simulink model "hover_model_estim_bsc_simple_v15"  (Simulink 7.1)
settings: Solver=ode45  StartTime=0.0  StopTime=200  RelTol=1e-4
values from neighbouring files (symbols this model uses):
  Am = [0 1 0 0 0 0;     0 0 0 0 0 0;     0 0 0 1 0 0;     0 0 0 0 0 0;     0 0 0 0 0 1;     0 0 0 0 0 0]    [Hover.m]    (also in Hoverparameter1.m = [0,1;0,0])
  Bm = [0 0 0 0;     -Kt/Jy -Kt/Jy Kt/Jy Kt/Jy;     0 0 0 0;     I*Kfn/Jp -I*Kfn/Jp 0 0;     0 0 0 0;     0 0 I*Kfc/Jr -I*Kfc/Jr]    [Hover.m]    (also in Hoverparameter1.m = [0,0,0,0;1,-1,0,0])
  Cm = [1 0 0 0 0 0;     0 0 1 0 0 0;     0 0 0 0 1 0]    [Hover.m]    (also in Hoverparameter1.m = [1,0])
  Ki = K(:,7:9)    [Hover.m]    (also in Hoverparameter1.m)
libraries: simulink x5, vrlib x1, simulink_extras x1
settings Model: Creator=user  LastModifiedBy=MorrisChen
settings DataIOCC: SignalLoggingName=sigsOut
settings OptimizationCC: InlineInvariantSignals=on
settings DebuggingCC: SaveWithParameterizedLinksMsg=none  SignalResolutionControl=TryResolveAllWithWarning  SolverPrmCheckMsg=none  MultiTaskDSMMsg=warning  MultiTaskCondExecSysMsg=none  StrictBusMsg=None
settings HardwareCC: TargetUnknown=on
settings RTWCC: IncludeERTFirstTime=on
settings GRTTargetCC: TargetFcnLib=ansi_tfl_tmw.mat

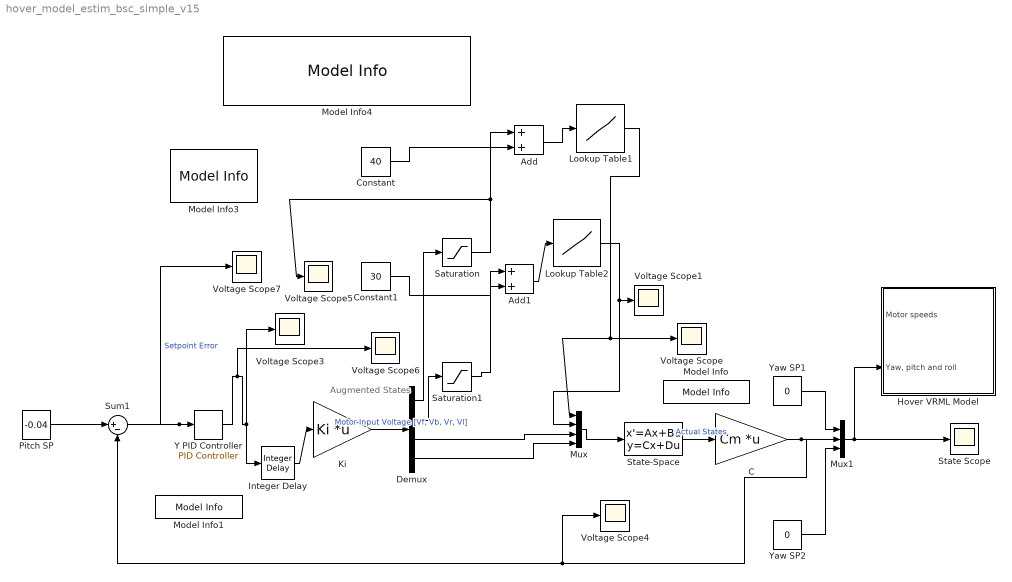
== system hover_model_estim_bsc_simple_v15 ==
  note: Augmented
      | States
  " Yaw SP1" : Constant  Value=0  OutDataType=sfix(16)  OutScaling=2^0
  " Yaw SP2" : Constant  Value=0  OutDataType=sfix(16)  OutScaling=2^0
  Add : Sum  OutDataType=sfix(16)  OutScaling=2^-10
  Add1 : Sum  OutDataType=sfix(16)  OutScaling=2^-10
  C : Gain  Gain=Cm  Multiplication=Matrix(K*u) (u vector)  ParameterDataType=sfix(16)  ParameterScaling=2^0  OutDataType=sfix(16)  OutScaling=2^0  SaturateOnIntegerOverflow=on  OutDataTypeStr=Inherit: Same as input  ParamDataTypeStr=Inherit: Same as input
  Constant : Constant  Value=40  OutDataType=sfix(16)  OutScaling=2^0
  Constant1 : Constant  Value=30  OutDataType=sfix(16)  OutScaling=2^0
  Demux : Demux
  Hover VRML Model : Subsystem
      mask Display: image(imread('3dofhover.jpg'))
  Integer Delay : simulink/Discrete/Integer Delay  vinit=0.0  samptime=-1  NumDelays=8
  Ki : Gain  Gain=Ki  Multiplication=Matrix(K*u) (u vector)  ParameterDataType=sfix(16)  ParameterScaling=2^0  OutDataType=sfix(16)  OutScaling=2^0  SaturateOnIntegerOverflow=on  OutDataTypeStr=Inherit: Same as input  ParamDataTypeStr=Inherit: Same as input
  Lookup Table1 : Lookup  InputValues="[0 74.99 75 79.99  80  84.99  85  89.99  90  94.99 95 99.99]"  Table="[0  0  6.62E-4  6.62E-4  6.62E-4  6.62E-4  7.5E-4  7.5E-4  1.0E-03  1.0E-03   1.0E-03  1.0E-03]"  OutDataType=sfix(16)  OutScaling=2^0
  Lookup Table2 : Lookup  InputValues="[0 74.99 75 79.99  80  84.99  85  89.99  90  94.99 95 99.99]"  Table="[0  0  1.2E-3  1.2E-3  1.2E-3 1.2E-3  1.2E-3  1.2E-3  1.2E-3  1.2E-3   1.4E-3  1.4E-3]"  OutDataType=sfix(16)  OutScaling=2^0
  Model Info : simulink/Model-Wide Utilities/Model Info  SystemSampleTime=-1  InitialBlockCM=None  BlockCM=None  Frame=on  DisplayStringWithTags=Plant  HorizontalTextAlignment=Center  LeftAlignmentValue=0.5  SourceBlockDiagram=hover_model_estim_bsc_simple_v15  TagMaxNumber=20
  Model Info1 : simulink/Model-Wide Utilities/Model Info  SystemSampleTime=-1  InitialBlockCM=None  BlockCM=None  Frame=on  DisplayStringWithTags=Controller  HorizontalTextAlignment=Center  LeftAlignmentValue=0.5  SourceBlockDiagram=hover_model_estim_bsc_simple_v15  TagMaxNumber=20
  Model Info3 : simulink/Model-Wide Utilities/Model Info  SystemSampleTime=-1  InitialBlockCM=None  BlockCM=None  Frame=on  DisplayStringWithTags=|  HorizontalTextAlignment=Center  LeftAlignmentValue=0.5  SourceBlockDiagram=hover_model_estim_bsc_simple_v15  TagMaxNumber=20
      | Command or
      | Reference
      | Input
  Model Info4 : simulink/Model-Wide Utilities/Model Info  SystemSampleTime=-1  InitialBlockCM=None  BlockCM=None  Frame=on  DisplayStringWithTags=|  HorizontalTextAlignment=Center  LeftAlignmentValue=0.5  SourceBlockDiagram=hover_model_estim_bsc_simple_v15  TagMaxNumber=20
      | This model is an observer based state controller
      | for the Quanser 3DOF Hover rig.
      | Written by B. Cazzolato 1/3/05.
      | Before this simulation can be run, you must
      | run the file "d_hover_bsc_new.m"
  Mux : Mux
  Mux1 : Mux  Inputs=3
  Pitch SP : Constant  Value=-0.04  OutDataType=sfix(16)  OutScaling=2^0
  Saturation : Saturate  UpperLimit=10000  LowerLimit=0  OutDataType=sfix(16)  OutScaling=2^0
  Saturation1 : Saturate  UpperLimit=10000  LowerLimit=0  OutDataType=sfix(16)  OutScaling=2^0
  State Scope : Scope
      settings: TimeRange=200  YMin=-0.085  YMax=0
  State-Space : StateSpace  A=Am  B=Bm  C=eye(2)  D=zeros(2,4)
  Sum1 : Sum  Inputs=|+-  OutDataType=sfix(16)  OutScaling=2^0  SaturateOnIntegerOverflow=on
  Voltage Scope{,1,3..7} (7 alike) : Scope
      Voltage Scope settings: YMin=0  YMax=0.001
      Voltage Scope1 settings: YMin=0  YMax=0.00035  SaveName=ScopeData2
      Voltage Scope3 settings: YMin=-2  YMax=6  SaveName=ScopeData4
      Voltage Scope4 settings: YMin=0  YMax=0.001  SaveName=ScopeData5  MaxDataPoints=50000
      Voltage Scope5 settings: YMin=-2  YMax=6  SaveName=ScopeData6
      Voltage Scope6 settings: YMin=-2  YMax=6  SaveName=ScopeData7
      Voltage Scope7 settings: YMin=-2  YMax=6  SaveName=ScopeData8
  Y PID Controller : simulink_extras/Additional Linear/PID Controller  SystemSampleTime=-1  P=40  I=0  D=40
  wires:
  State-Space/1 -> C/1  "Actual States"
  Pitch SP/1 -> Sum1/1
  Sum1/1 -> Y PID Controller/1, Voltage Scope7/1  "Setpoint Error"
  C/1 -> Mux1/2, Sum1/2, Voltage Scope4/1
  " Yaw SP1"/1 -> Mux1/1
  " Yaw SP2"/1 -> Mux1/3
  Mux1/1 -> Hover VRML Model/2("Yaw, pitch and roll"), State Scope/1
  Y PID Controller/1 -> Integer Delay/1, Voltage Scope3/1, Voltage Scope6/1
  Integer Delay/1 -> Ki/1
  Demux/1 -> Saturation/1
  Demux/2 -> Saturation1/1
  Ki/1 -> Demux/1  "Motor Input Voltage [Vf, Vb, Vr, Vl]"
  Demux/3 -> Mux/3
  Demux/4 -> Mux/4
  Mux/1 -> State-Space/1
  Saturation/1 -> Add/1, Voltage Scope5/1
  Saturation1/1 -> Add1/1
  Lookup Table2/1 -> Voltage Scope1/1, Mux/2
  Lookup Table1/1 -> Mux/1, Voltage Scope/1
  Constant/1 -> Add/2
  Add/1 -> Lookup Table1/1
  Constant1/1 -> Add1/2
  Add1/1 -> Lookup Table2/1

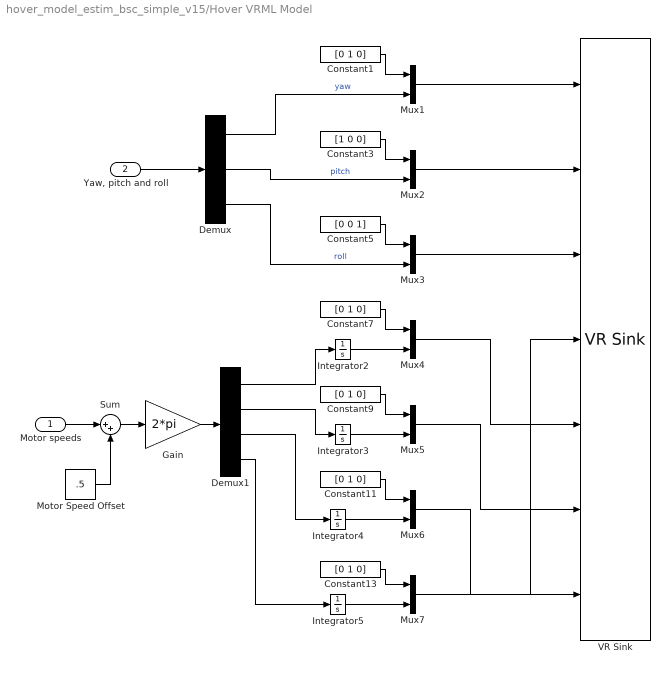
== system hover_model_estim_bsc_simple_v15/Hover VRML Model ==
  Motor speeds : Inport  OutDataType=sfix(16)  OutScaling=2^0
  "Yaw, pitch and roll" : Inport  Port=2  OutDataType=sfix(16)  OutScaling=2^0
  Constant{1,7,9,11,13} (5 alike) : Constant  Value=[0 1 0]  OutDataType=sfix(16)  OutScaling=2^0
  Constant3 : Constant  Value=[1 0 0]  OutDataType=sfix(16)  OutScaling=2^0
  Constant5 : Constant  Value=[0 0 1]  OutDataType=sfix(16)  OutScaling=2^0
  Demux : Demux  Outputs=3
  Demux1 : Demux
  Gain : Gain  Gain=2*pi  ParameterDataType=sfix(16)  ParameterScaling=2^0  OutDataType=sfix(16)  OutScaling=2^0
  Integrator{2..5} (4 alike) : Integrator
  Motor Speed Offset : Constant  Value=.5  OutDataType=sfix(16)  OutScaling=2^0
  Mux{1..7} (7 alike) : Mux  Inputs=2
  Sum : Sum  Inputs=|++  OutDataType=sfix(16)  OutScaling=2^0
  VR Sink : vrlib/VR Sink  SampleTime=0.02  ViewEnable=on  RemoteChange=off  RemoteView=off  FieldsWritten=YAW.rotation.4.1.double#PITCH.rotation.4.1.double#ROLL.rotation.4.1.double#LEFT_PROP.rotation.4.1.double#FRONT_PROP.rotation.4.1.double#BACK_PROP.rotation.4.1.double#RIGHT_PROP.rotation.4.1.double  WorldFileName=THREEDOF_SIMULINK.WRL  AutoView=off  VideoDimensions=[]  FigureProperties="{'Position', 'Name', 'Viewpoint', 'CameraBound', 'CameraDirection', 'CameraPosition', 'CameraUpVector', 'ZoomFactor', 'Antialiasing', 'Headlight', 'Lighting', 'NavPanel', 'StatusBar', 'ToolBar', 'Textures', 'Transparency', 'Wireframe', 'NavZones', 'NavMode', 'NavSpeed', 'Record2DCompressMethod', 'Record2DCompressQuality', 'Record2D', 'Record2DFileName', 'Record2DFPS'; [5.0000000000000000e+000  9.2000000000000000e+001  5.7600000000000000e+002  3.8000000000000000e+002], '', 'FRONT', 'on', [0.0000000000000000e+000  0.0000000000000000e+000 -1.0000000000000000e+000], [0.0000000000000000e+000  0.0000000000000000e+000  0.0000000000000000e+000], [0.0000000000000000e+000  1.0000000000000000e+000  0.0000000000000000e+000], [1.0000000000000000e+000], 'off', 'on', 'on', 'halfbar', 'on', 'on', 'on', 'on', 'off', 'off', 'fly', 'normal', 'auto', [7.5000000000000000e+001], 'off', '%f_anim_%n.avi', [1.5000000000000000e+001]}"
  wires:
  Constant1/1 -> Mux1/1
  Constant3/1 -> Mux2/1
  Constant5/1 -> Mux3/1
  Constant7/1 -> Mux4/1
  Constant9/1 -> Mux5/1
  Constant11/1 -> Mux6/1
  Constant13/1 -> Mux7/1
  Integrator2/1 -> Mux4/2
  Integrator3/1 -> Mux5/2
  Integrator4/1 -> Mux6/2
  Integrator5/1 -> Mux7/2
  Demux/1 -> Mux1/2  "yaw"
  Demux/3 -> Mux3/2  "roll"
  Demux1/1 -> Integrator2/1
  Demux1/2 -> Integrator3/1
  Demux1/3 -> Integrator4/1
  "Yaw, pitch and roll"/1 -> Demux/1
  Demux/2 -> Mux2/2  "pitch"
  Demux1/4 -> Integrator5/1
  Gain/1 -> Demux1/1
  Sum/1 -> Gain/1
  Motor speeds/1 -> Sum/1
  Motor Speed Offset/1 -> Sum/2
  Mux1/1 -> VR Sink/1
  Mux2/1 -> VR Sink/2
  Mux3/1 -> VR Sink/3
  Mux4/1 -> VR Sink/5
  Mux5/1 -> VR Sink/6
  Mux6/1 -> VR Sink/7
  Mux7/1 -> VR Sink/4
